simulink model "chap6_2sim"  (Simulink 3.00)
settings: Solver=ode45  StartTime=0.0  StopTime=5  RelTol=1e-3
settings Model: LastModifiedBy=liu

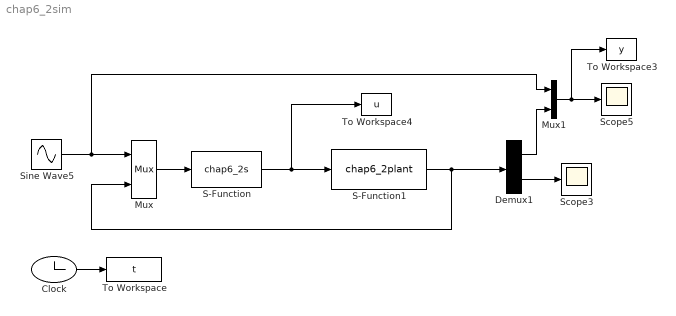
== system chap6_2sim ==
  Clock : Clock
  Demux1 : Demux  Outputs=2
  Mux : Mux  Inputs=2
      settings: DisplayOption=none
  Mux1 : Mux  Inputs=2
  S-Function : S-Function  FunctionName=chap6_2s  PortCounts=[]  SFunctionModules=''
  S-Function1 : S-Function  FunctionName=chap6_2plant  PortCounts=[]  SFunctionModules=''
  Scope3 : Scope
      settings: TimeRange=auto  YMin=-0.15  YMax=0.325  SaveToWorkspace=off  SaveName=ScopeData
  Scope5 : Scope
      settings: TimeRange=auto  YMin=-1  YMax=1  SaveToWorkspace=off  SaveName=ScopeData  MaxRows=50000
  Sine Wave5 : Sin  Amplitude=1  Frequency=2*pi  Phase=0  SampleTime=0
  To Workspace : ToWorkspace  VariableName=t  SampleTime=-1  SaveFormat=Matrix
  To Workspace3 : ToWorkspace  VariableName=y  SampleTime=-1  SaveFormat=Matrix
  To Workspace4 : ToWorkspace  VariableName=u  SampleTime=-1  SaveFormat=Matrix
  wires:
  Mux/1 -> S-Function/1
  S-Function/1 -> S-Function1/1, To Workspace4/1
  S-Function1/1 -> Mux/2, Demux1/1
  Demux1/1 -> Mux1/2
  Sine Wave5/1 -> Mux/1, Mux1/1
  Demux1/2 -> Scope3/1
  Mux1/1 -> Scope5/1, To Workspace3/1
  Clock/1 -> To Workspace/1
